simulink model "flexibleMissileFullIO"  (R2014a)
settings: Solver=ode45  StartTime=0.0  StopTime=10.0  MaxStep=0.2  RelTol=1e-3
values from neighbouring files (symbols this model uses):
  CLd = pi*ARf*Sfins/(1+sqrt(1+(pi*ARf/(2*0.7))^2))/S    [loadModel_EB.m]
  rho = 1.21    [loadModel_EB.m]
  S = pi*D_booster^4/4    (= 0.0131916732161)    [loadModel_EB.m]
  Vx = M*sqrt(gamma_air*r*T)    [loadModel_EB.m]
libraries: RCTblocks x2
settings Model: Creator=s220385  LastModifiedBy=s220385
settings OptimizationCC: SimCompilerOptimization=off
settings DebuggingCC: MergeDetectMultiDrivingBlocksExec=error  FrameProcessingCompatibilityMsg=error
settings RTWCC: RTWCompilerOptimization=off

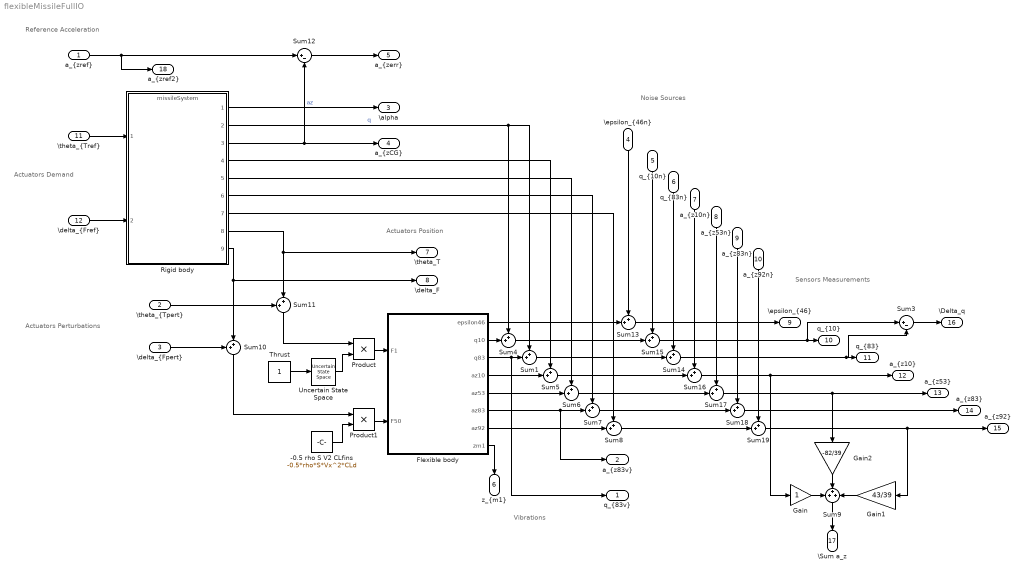
== system flexibleMissileFullIO ==
  note: Noise Sources
  note: Sensors Measurements
  note: Reference Acceleration
  note: Actuators Demand
  note: Actuators Position
  note: Actuators Perturbations
  note: Vibrations
  "a_{zref}" : Inport
  "\\theta_{Tpert}" : Inport  Port=2
  "\\delta_{Fpert}" : Inport  Port=3
  "\\epsilon_{46n}" : Inport  Port=4
  "q_{10n}" : Inport  Port=5
  "q_{83n}" : Inport  Port=6
  "a_{z10n}" : Inport  Port=7
  "a_{z53n}" : Inport  Port=8
  "a_{z83n}" : Inport  Port=9
  "a_{z92n}" : Inport  Port=10
  "\\theta_{Tref}" : Inport  Port=11
  "\\delta_{Fref}" : Inport  Port=12
  -0.5 rho S V2 CLfins : Constant  Value=-0.5*rho*S*Vx^2*CLd
  Flexible body : Subsystem
      mask Display:
      | port_label('input',1,'Tail Lateral Force')
      | port_label('input',2,'Fins Lateral Force')
      | 
      | port_label('output',1,'\epsilon_{46}','texmode','on')
      | port_label('output',2,'q_{10}','texmode','on')
      | port_label('output',3,'q_{83}','texmode','on')
      | port_label('output',4,'a_{z10}','texmode','on')
      | port_label('output',5,'a_{z53}','texmode','on')
      | port_label('output',6,'a_{z83}','texmode','on')
      | port_label('output',7,'a_{z92}','texmode','on')
      | port_label('output',8,'z_{m1}','texmode','on')
  Gain : Gain
  Gain1 : Gain  Gain=43/39
  Gain2 : Gain  Gain=-82/39
  Product : Product
  Product1 : Product
  Rigid body : ModelReference  ModelNameDialog=missileSystem  SimulationMode=Normal  ModelReferenceVersion=1.18  CopyOfModelName=missileSystem  DefaultDataLogging=on
      mask Display:
      | port_label('input',1,'\theta_{Tref}','texmode','on')
      | port_label('input',2,'\delta_{Fref}','texmode','on')
      | 
      | port_label('output',1,'\alpha','texmode','on')
      | port_label('output',2,'q','texmode','on')
      | port_label('output', 3, 'a_{zCG}','texmode','on')
      | port_label('output', 4, 'a_{z10}','texmode','on')
      | port_label('output', 5, 'a_{z53}','texmode','on')
      | port_label('output', 6, 'a_{z83}','texmode','on')
      | port_label('output', 7, 'a_{z91}','texmode','on')
      | port_label('output',8,'\theta_T','texmode','on')
      | port_label('output',9,'\delta_F','texmode','on')
  Sum{1,4..8,10..11,13..19} (15 alike) : Sum  Inputs=++|
  Sum12 : Sum  Inputs=|+-
  Sum3 : Sum  Inputs=|+-
  Sum9 : Sum  Inputs=+++
  Thrust : Constant
  Uncertain State Space : RCTblocks/Uncertain State Space  Tag=USS  USystem=T0  UValue=[]  X0=[]  uX0=[]
  "q_{83v}" : Outport
  "a_{z83v}" : Outport  Port=2
  \alpha : Outport  Port=3
  "a_{zCG}" : Outport  Port=4
  "a_{zerr}" : Outport  Port=5
  "z_{m1}" : Outport  Port=6
  \theta_T : Outport  Port=7
  \delta_F : Outport  Port=8
  "\\epsilon_{46}" : Outport  Port=9
  "q_{10}" : Outport  Port=10
  "q_{83}" : Outport  Port=11
  "a_{z10}" : Outport  Port=12
  "a_{z53}" : Outport  Port=13
  "a_{z83}" : Outport  Port=14
  "a_{z92}" : Outport  Port=15
  \Delta_q : Outport  Port=16
  \Sum a_z : Outport  Port=17
  "a_{zref2}" : Outport  Port=18
  wires:
  Product/1 -> Flexible body/1(F1)
  Thrust/1 -> Uncertain State Space/1
  "\\theta_{Tref}"/1 -> Rigid body/1
  Rigid body/1 -> \alpha/1
  Flexible body/3(q83) -> "q_{83v}"/1, Sum1/2
  Flexible body/4(az10) -> Sum5/2
  Flexible body/5(az53) -> Sum6/2
  Flexible body/6(az83) -> "a_{z83v}"/1, Sum7/2
  Flexible body/7(az92) -> Sum8/2
  Flexible body/2(q10) -> Sum4/2
  Rigid body/2 -> Sum4/1, Sum1/1  "q"
  Rigid body/4 -> Sum5/1
  Rigid body/5 -> Sum6/1
  Rigid body/6 -> Sum7/1
  Rigid body/7 -> Sum8/1
  Rigid body/3 -> Sum12/2, "a_{zCG}"/1  "az"
  "\\delta_{Fref}"/1 -> Rigid body/2
  Rigid body/9 -> Sum10/2, \delta_F/1
  Sum10/1 -> Product1/1
  Product1/1 -> Flexible body/2(F50)
  -0.5 rho S V2 CLfins/1 -> Product1/2
  Sum3/1 -> \Delta_q/1
  Sum9/1 -> \Sum a_z/1
  Gain/1 -> Sum9/1
  Gain1/1 -> Sum9/3
  Gain2/1 -> Sum9/2
  Uncertain State Space/1 -> Product/2
  "\\delta_{Fpert}"/1 -> Sum10/1
  "\\theta_{Tpert}"/1 -> Sum11/1
  Sum11/1 -> Product/1
  "a_{zref}"/1 -> "a_{zref2}"/1, Sum12/1
  Sum12/1 -> "a_{zerr}"/1
  Flexible body/8(zm1) -> "z_{m1}"/1
  Sum8/1 -> Sum19/2
  "q_{10n}"/1 -> Sum15/1
  "q_{83n}"/1 -> Sum14/1
  "a_{z10n}"/1 -> Sum16/1
  "a_{z53n}"/1 -> Sum17/1
  "a_{z83n}"/1 -> Sum18/1
  "a_{z92n}"/1 -> Sum19/1
  Sum4/1 -> Sum15/2
  Sum1/1 -> Sum14/2
  Sum5/1 -> Sum16/2
  Sum6/1 -> Sum17/2
  Sum7/1 -> Sum18/2
  Sum15/1 -> Sum3/1, "q_{10}"/1
  Flexible body/1(epsilon46) -> Sum13/2
  Sum13/1 -> "\\epsilon_{46}"/1
  "\\epsilon_{46n}"/1 -> Sum13/1
  Sum14/1 -> Sum3/2, "q_{83}"/1
  Sum16/1 -> Gain/1, "a_{z10}"/1
  Sum17/1 -> Gain2/1, "a_{z53}"/1
  Sum18/1 -> "a_{z83}"/1
  Sum19/1 -> Gain1/1, "a_{z92}"/1
  Rigid body/8 -> \theta_T/1, Sum11/2

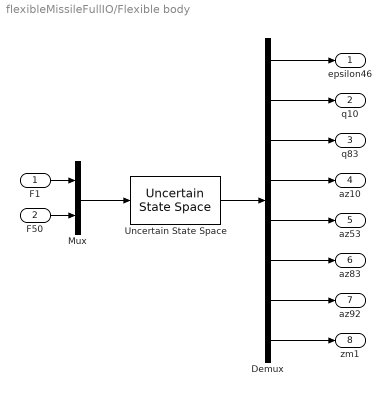
== system flexibleMissileFullIO/Flexible body ==
  F1 : Inport
  F50 : Inport  Port=2
  Demux : Demux  Outputs=8
  Mux : Mux  Inputs=2
  Uncertain State Space : RCTblocks/Uncertain State Space  Tag=USS  USystem=flexi  UValue=[]  X0=[]  uX0=[]
  epsilon46 : Outport
  q10 : Outport  Port=2
  q83 : Outport  Port=3
  az10 : Outport  Port=4
  az53 : Outport  Port=5
  az83 : Outport  Port=6
  az92 : Outport  Port=7
  zm1 : Outport  Port=8
  wires:
  Demux/1 -> epsilon46/1
  Demux/2 -> q10/1
  Demux/3 -> q83/1
  Demux/4 -> az10/1
  Demux/5 -> az53/1
  Demux/6 -> az83/1
  Demux/7 -> az92/1
  F1/1 -> Mux/1
  F50/1 -> Mux/2
  Uncertain State Space/1 -> Demux/1
  Demux/8 -> zm1/1
  Mux/1 -> Uncertain State Space/1
